simulink model "rtlsdr_datafm_image_audio_Added_Noise"  (R2019a)
settings: Solver=ode45  StartTime=0.0  StopTime=170  RelTol=1e-3  EnableMultiTasking=on
PreLoadFcn:
  | %%%%%%%%%%%%%%%%%%%%%%%%%%%%%%%%%%%%%%%%%%%%%%%%%%%%%%%%%%%%%%%%%%%%%%%%%%%
  | % check to see if Simulink library folder is missing from the MATLAB path %
  | %%%%%%%%%%%%%%%%%%%%%%%%%%%%%%%%%%%%%%%%%%%%%%%%%%%%%%%%%%%%%%%%%%%%%%%%%%%
  | if isempty(strfind(path, 'rtlsdr_book_library'))
  | 
  |     % create error window
  |     fig_error = figure(...
  |         'Name', 'Error: RTL-SDR Book Library',...
  |         'Toolbar','none',...
  |         'MenuBar','none',...
  |         'NumberTitle','off',...
  |         'Resize','off',...
  |         'WindowStyle','modal');
  |     fig_error.Position(3) = 600;
  |     fig_error.Position(4) = 150;
  |     fig_axes = axes(...
  |         'Parent',fig_error,...
  |         'Position',[0,0,1,1],...
  |         'visible','off');
  |     % error message
  |     t_title = text(.05,.8,...
  |         'MISSING DIRECTORIES',...
  |         'FontSize',11.5);
  |     t_body = text(.075,.6,...
  |         [{'Simulink cannot find the  \it{<root>}\rm / \it{rtlsdr\_book\_library}\rm  folder in the \it{MATLAB Path}\rm.'},...
  |         {'Please set the MATLAB path following the instructions given in Exercise 2.4.'}],...
  |         'FontSize',10.5);
  |     % buttons
  |     btn_path = uicontrol(...
  |         'Parent',fig_error,...
  |         'String','Set Path Now',...
  |         'FontSize',10,...
  |         'Callback', 'pathtool; close(fig_error);',...
  |         'Position', [fig_error.Position(3)/2-210, 30, 200, 30]);
  |     btn_abort = uicontrol(...
  |         'Parent',fig_error,...
  |         'String','No thanks',...
  |         'FontSize',10,...
  |         'Callback', 'close(fig_error); abort=1;',...
  |         'Position', [fig_error.Position(3)/2+10, 30, 200, 30]);
  | 
  |     % pause to allow user to interact with error box
  |     uiwait(fig_error);
  | 
  |     % abort simulation
  |     try
  |         if abort==1
  |             set_param(gcs, 'SimulationCommand', 'stop');
  |         end
  |     end
  | 
  |     % if user has set path, allow diagram to be updated
  |     if ~exist('abort','var')
  |         % create error window
  |         fig_update = figure(...
  |             'Name', 'Update Diagram',...
  |             'Toolbar','none',...
  |             'MenuBar','none',...
  |             'NumberTitle','off',...
  |             'Resize','off');
  |         fig_update.Position(3) = 400;
  |         fig_update.Position(4) = 120;
  |         fig_axes = axes(...
  |             'Parent',fig_update,...
  |             'Position',[0,0,1,1],...
  |             'visible','off');
  |         % instruction message
  |         t_body = text(.075,.7,...
  |             'Once you have set the path, update the block diagram',...
  |             'FontSize',10.5);
  |         % button
  |         btn_update = uicontrol(...
  |             'Parent',fig_update,...
  |             'String','Update Block Diagram',...
  |             'FontSize',10,...
  |             'Callback', 'set_param(gcs,''SimulationCommand'',''update''); close(gcf)',...
  |             'Position', [fig_update.Position(3)/2-100, 30, 200, 30]);
  |     end
  | 
  |     % clear error components
  |     clear('fig_error','fig_update','fig_axes','t_title','t_body','btn_path','btn_abort','btn_update','abort');
  | 
  | end
  | %%%%%%%%%%%%%%%%%%%%%%%%%%%%%%%%%%%%%%%%%%%%%%%%%%%%%%%%%%%%%%%%%%%%%%%%%%%
undefined symbols (not defined in the file): dfilt, fdesignblkfcn, frm, gcbh, startfcn_spectrum_analyzer
libraries: dsparch4 x3, simulink x3, dspmlti4 x2, commutil2 x2, simulink_need_slupdate x2, rtlsdr_book_library x2, commrfcorlib x1, commchan3 x1, dspstat3 x1, dspfdesign x1, sdrrlib x1, dspobslib x1
CloseFcn:
  | closefcn_model;
Description:
  | Software, Simulation Examples and Design Exercises Licence Agreement
  | 
  | This license agreement refers to the simulation examples, design exercises and files,
  | and associated software MATLAB and Simulink resources that accompany the book:
  | 
  |      Title: Software Defined Radio using MATLAB & Simulink and the RTL-SDR
  |      Published by Strathclyde Academic Media, 2015
  |      Authored by Robert W. Stewart, Kenneth W. Barlee, Dale S.W. Atkinson,
  |      and Louise H. Crockett
  | 
  | and made available as a download from, www.desktopSDR.com or variously acquired
  | by other means such as via USB storage, cloud storage, disk or any other electronic
  | or optical or magnetic storage mechanism. These files and associated software may
  | be used subject to the terms of agreement of the conditions below:
  | 
  |     Copyright © 2015 Robert W. Stewart, Kenneth W. Barlee, Dale S.W. Atkinson,
  |     and Louise H. Crockett
  |     All rights reserved.
  | 
  | Redistribution and use in source and binary forms, with or without modification, are
  | permitted provided that the following conditions are met:
  | 
  |    1.  Redistributions of source code must retain the above copyright notice, this list of
  |         conditions and the following disclaimer.
  | 
  |    2.  Redistributions in binary form must reproduce the above copyright notice, this
  |         list of conditions and the following disclaimer in the documentation and/or other
  |         materials provided with the distribution.
  | 
  |    3.  Neither the name of the copyright holder nor the names of its contributors may
  |         be used to endorse or promote products derived from this software without
  |         specific prior written permission.
  | 
  |    4.  In all cases, the software is, and all modifications and derivatives of the
  |         software shall be, licensed to you solely for use in conjunction with The
  |         MathWorks, Inc. products and service offerings.
  | 
  | THIS SOFTWARE IS PROVIDED BY THE COPYRIGHT HOLDERS AND CONTRIBUTORS
  | "AS IS" AND ANY EXPRESS OR IMPLIED WARRANTIES, INCLUDING, BUT NOT LIMITED
  | TO, THE IMPLIED WARRANTIES OF MERCHANTABILITY AND FITNESS FOR A
  | PARTICULAR PURPOSE ARE DISCLAIMED. IN NO EVENT SHALL THE COPYRIGHT
  | HOLDER OR CONTRIBUTORS BE LIABLE FOR ANY DIRECT, INDIRECT, INCIDENTAL,
  | SPECIAL, EXEMPLARY, OR CONSEQUENTIAL DAMAGES (INCLUDING, BUT NOT
  | LIMITED TO, PROCUREMENT OF SUBSTITUTE GOODS OR SERVICES; LOSS OF USE,
  | DATA, OR PROFITS; OR BUSINESS INTERRUPTION) HOWEVER CAUSED AND ON ANY
  | THEORY OF LIABILITY, WHETHER IN CONTRACT, STRICT LIABILITY, OR TORT
  | (INCLUDING NEGLIGENCE OR OTHERWISE) ARISING IN ANY WAY OUT OF THE USE
  | OF THIS SOFTWARE, EVEN IF ADVISED OF THE POSSIBILITY OF SUCH DAMAGE.
  | 
  | 
  | Audio Tracks used in Simulations Examples and Design Exercises
  | 
  | The music and vocal files used within the Examples files and software within the book
  | were variously written, arranged, performed, recorded and produced by Garrey Rice,
  | Adam Struth, Jamie Struth, Iain Thistlethwaite and also Marshall Craigmyle who
  | collectively, and individually where appropriate, assert and retain all of their copyright,
  | performance and artistic rights. Permission to use and reproduce this music is
  | granted for all purposes associated with MATLAB and Simulink software and the
  | simulation examples and design exercises files that accompany this book. Requests to
  | use the music for any other purpose should be directed to: info@desktopSDR.com.
  | For information on music track names, full credits, and links to the musicians please
  | refer to www.desktopSDR.com/more/audio.
settings Model: ModifiedByFormat=desktopSDR Team  SimulationMode=accelerator  Creator=desktopSDR Team  LastModifiedBy=desktopSDR Team
settings DataIOCC: SaveFormat=Array  SaveOutput=off  SignalLogging=off  SaveTime=off  ReturnWorkspaceOutputs=off
settings OptimizationCC: LifeSpan=inf
settings DebuggingCC: SolverPrmCheckMsg=warning  AllowSymbolicDim=off  SFUnexpectedBacktrackingDiag=warning  SFNoUnconditionalDefaultTransitionDiag=warning  SFExecutionAtInitializationDiag=none  ArithmeticOperatorsInVariantConditions=warning
settings HardwareCC: ProdBitPerPointer=32  ProdBitPerSizeT=32  ProdBitPerPtrDiffT=32  ProdLargestAtomicFloat=None  ProdIntDivRoundTo=Undefined  ProdEndianess=Unspecified  ProdWordSize=32  ProdHWDeviceType=32-bit Generic
settings ModelReferenceCC: PropagateSignalLabelsOutOfModel=off
settings SFSimCC: SimUseLocalCustomCode=off
settings RTWCC: RTWUseLocalCustomCode=off
settings CodeAppCC: StateflowObjectComments=on
settings GRTTargetCC: TargetLangStandard=C89/C90 (ANSI)  GeneratePreprocessorConditionals=Disable all
settings ConfigComp: CovMetricSettings=dw  CovHtmlReporting=on  CovSaveCumulativeToWorkspaceVar=on  CovSaveSingleToWorkspaceVar=on  CovExternalEMLEnable=off  CovSFcnEnable=off

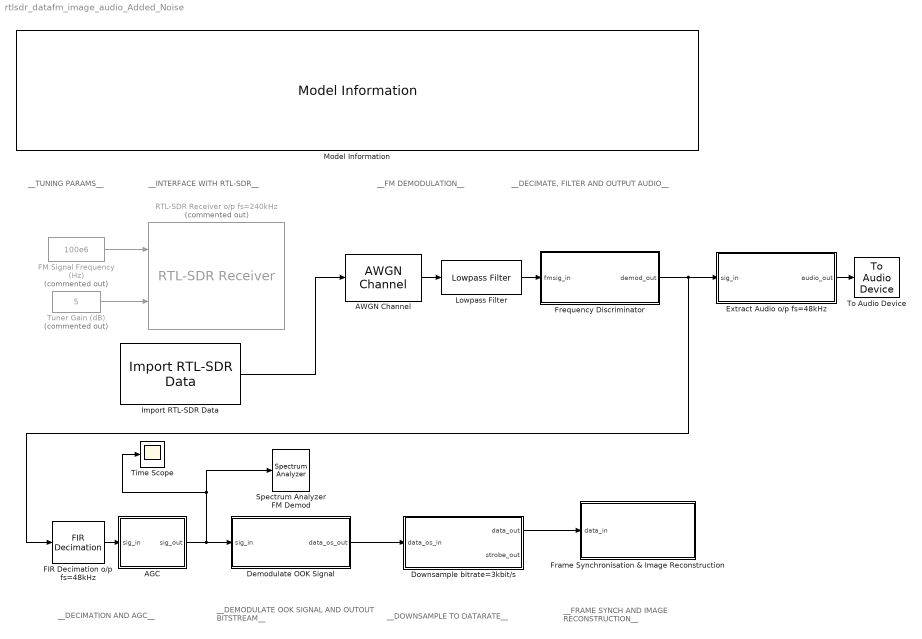
== system rtlsdr_datafm_image_audio_Added_Noise ==
  note: __FRAME SYNCH AND
      | IMAGE RECONSTRUCTION__
  note: __FM DEMODULATION__
  note: __INTERFACE WITH RTL-SDR__
  note: __TUNING PARAMS__
  note: __DECIMATE, FILTER AND OUTPUT AUDIO__
  note: __DECIMATION AND AGC__
  note: __DOWNSAMPLE TO DATARATE__
  note: __DEMODULATE OOK SIGNAL
      | AND OUTOUT BITSTREAM__
  AGC : Subsystem
  AWGN Channel : commchan3/AWGN Channel  InputProcessing=Columns as channels (frame based)  seed=67  noiseMode="Signal to noise ratio  (SNR)"  EbNodB=10  EsNodB=10  SNRdB=10  bitsPerSym=1  Ps=1  Tsym=1  variance=1
      settings: SourceProductName=Communications Toolbox
  Demodulate OOK Signal : Subsystem
  Downsample bitrate=3kbit/s : Subsystem  mask{fs=3e3}
      mask prompts: fs "Data bitrate (bit/s):"
      mask help: This block is used to downsample the received (oversampled) data back to its original bitrate. It comprises of an edge detector and a sampler.
      mask DialogControl DescGroupVar Prompt: Downsampler for Data in FM Signal
  Extract Audio o/p fs=48kHz : Subsystem
  FIR Decimation o/p fs=48kHz : dspmlti4/FIR Decimation  FilterSource=Dialog parameters  h=firpm(150, [0 15e3 20e3 (240e3/2)]/(240e3/2), [1 1 0 0], [1 1],20)  D=5  filtStruct=Direct form  FilterObject=Hm_firdecim  InputProcessing=Columns as channels (frame based)  framing=Allow multirate processing  inputOffset=0  outputBufInitCond=0  roundingMode=Floor  overflowMode=off  firstCoeffDataTypeStr=Inherit: Same word length as input  firstCoeffMin=[]  firstCoeffMax=[]  firstCoeffLastDataTypeStr=Inherit: Same word length as input  outputDataTypeStr=Inherit: Same as accumulator  outputMin=[]  outputMax=[]  outputLastDataTypeStr=Inherit: Same as accumulator
  "FM Signal Frequency (Hz) " : Constant  Commented=on  Value=100e6
  Frame Synchronisation & Image Reconstruction : Subsystem  mask(Receiver Parameter Settings){binary_len=8}
      mask prompts: binary_len "Image Pixel Bit Depth"
      mask help: The subsystem implements frame synchronisation to re-frame the received data back to its original frame structure. The preamble is then removed before the remaining header and payload data are used to recover and reconstruct the transmitted image.
      mask init:
      | try 
      |     image_receive;
      | catch ME
      |     if(strcmp(ME.identifier,'MATLAB.UndefinedFunction'))
      |         error('Unable to find "image_receive.m".');
      |     end
      |     rethrow(ME);
      | end
      mask Callback binary_len:
      | try
      |     image_receive;
      | end
  Frequency Discriminator : Subsystem
  Import RTL-SDR Data : rtlsdr_book_library/Additional Tools/Import RTL-SDR Data  filename=datafm_image_audio.mat  frm_size=4096  data_type=single
      settings: SourceProductName=RTL-SDR Book Library
  Lowpass Filter : dspfdesign/Lowpass Filter  FilterType=FIR  DesignForMinimumOrder=on  FilterOrder=50  PassbandFrequency=5e3  StopbandFrequency=80e3  PassbandRipple=0.1  StopbandAttenuation=80  InheritSampleRate=off  SampleRate=240e3  SimulateUsing=Interpreted execution  roundingMode=Floor  coeffsDataTypeStr=fixdt(1,16)
  Model Information : rtlsdr_book_library/Additional Tools/Model Information/Model Information
      settings: SourceProductName=RTL-SDR Book Library
  RTL-SDR Receiver o/p fs=240kHz : sdrrlib/RTL-SDR Receiver  Commented=on  IPAddress=0  CenterFrequencySource=Input port  CenterFrequency=433.9e6  GainSource=Input port  Gain=15  ADCRate=240e3  FrequencyCorrection=0  LostSamplesOutputPort=off  LatencyOutputPort=off  OutputDataType=single  FrameLength=4096  EnableBurstMode=off  NumFramesInBurst=20  sobjType=sdrr.internal.SDRRTLReceiverSL  dataUDPPort=-1  ctrlUDPPort=-1  subDeviceList=nosubdev  sdrBlockType=SDRBlockTypeSLT.SDRRxBlock  requester=UNUSED_BY_SFCN  sdrExecutionMode=SDRExecutionModeSLT.ExecModeHW  BypassUserLogic=off  DecimatorSelect=DDC decimator  SourceSelect=RF data  SineAmplitude=16000  EnableInternalClock=off  BypassIQBalance=off  IFBandwidth=40e6  ADCRateSource=Dialog  IntermediateFrequency=0  DecimationFactorSource=Dialog  DecimationFactor=512  RFFrequencyIsTunable=logical(1)  SampleTime=(4096)/(240e3)  IFBandwidthSource=Dialog  SineFrequency=30000  BypassDCBlockingFilter=off  IntermediateFrequencySource=Dialog  IQBalanceCoefficients=64  SkipAllHardwareResetAndInitialization=off  EnableIQCalibrationTable=on  CacheIQCalibrationTable=off  EnableOffsetTuning=off  EnableRTLAGC=off  EnableTestMode=off  EnableTunerAGC=off  FrequencyCorrectionSource=Dialog  NumMLBuffers=128  NumUSBBuffers=16  RTLCrystalFrequency=28800000  TunerCrystalFrequency=28800000
      settings: SourceProductName=Communications Toolbox Support Package for RTL-SDR Radio  SourceProductBaseCode=RTLSDR
  Spectrum Analyzer FM Demod : SpectrumAnalyzer  StartFcn=startfcn_spectrum_analyzer;
  Time Scope : Scope
      settings: StartFcn=startfcn_time_scope
  To Audio Device : dspobslib/To Audio Device  deviceName=Default  inheritSampleRate=on  sampleRate=44100  deviceDatatype=Determine from input data type  autoBufferSize=on  bufferSize=4096  queueDuration=1.0  defaultOutputChannelMapping=on  outputChannelMapping=1:2  outputNumUnderrunSamples=off
      settings: SourceProductName=DSP System Toolbox  SourceProductBaseCode=DS
  Tuner Gain (dB) : Constant  Commented=on  Value=5
  wires:
  Tuner Gain (dB)/1 -> RTL-SDR Receiver o/p fs=240kHz/2
  "FM Signal Frequency (Hz) "/1 -> RTL-SDR Receiver o/p fs=240kHz/1
  Extract Audio o/p fs=48kHz/1(audio_out) -> To Audio Device/1
  Downsample bitrate=3kbit/s/1(data_out) -> Frame Synchronisation & Image Reconstruction/1(data_in)
  FIR Decimation o/p fs=48kHz/1 -> AGC/1(sig_in)
  Frequency Discriminator/1(demod_out) -> Extract Audio o/p fs=48kHz/1(sig_in), FIR Decimation o/p fs=48kHz/1
  Demodulate OOK Signal/1(data_os_out) -> Downsample bitrate=3kbit/s/1(data_os_in)
  AGC/1(sig_out) -> Demodulate OOK Signal/1(sig_in), Time Scope/1, Spectrum Analyzer FM Demod/1
  AWGN Channel/1 -> Lowpass Filter/1
  Import RTL-SDR Data/1 -> AWGN Channel/1
  Lowpass Filter/1 -> Frequency Discriminator/1(fmsig_in)

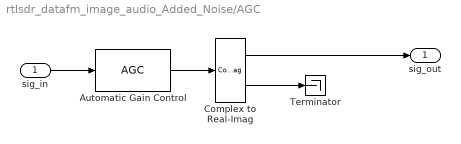
== system rtlsdr_datafm_image_audio_Added_Noise/AGC ==
  sig_in : Inport
  Automatic Gain Control : commrfcorlib/AGC  LegacyMode=off  DetectorMethod=Rectifier  LoopMethod=Linear  UpdatePeriod=128  StepSize=0.03  AdaptationStepSize=(0.03)/(128)  DesiredOutputPower=1  AveragingLength=128  MaximumGain=20  MaxPowerGain=20  GainOutputPort=off  InputPowerOutputPort=off  SimulateUsing=Code generation
      settings: SourceProductName=Communications Toolbox
  Complex to Real-Imag : ComplexToRealImag
  Terminator : Terminator
  sig_out : Outport
  wires:
  Complex to Real-Imag/1 -> sig_out/1
  Automatic Gain Control/1 -> Complex to Real-Imag/1
  sig_in/1 -> Automatic Gain Control/1
  Complex to Real-Imag/2 -> Terminator/1

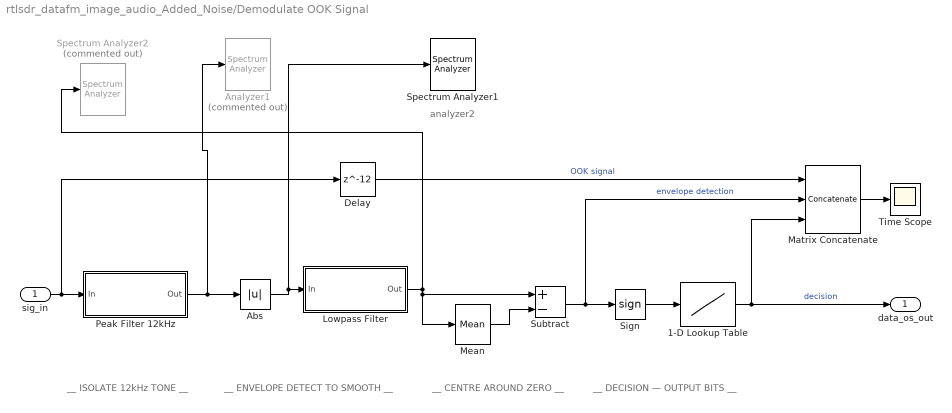
== system rtlsdr_datafm_image_audio_Added_Noise/Demodulate OOK Signal ==
  note: analyzer2
  note: __ ISOLATE 12kHz TONE __
  note: __ ENVELOPE DETECT TO SMOOTH __
  note: __ CENTRE AROUND ZERO __
  note: __ DECISION — OUTPUT BITS __
  sig_in : Inport
  " Analyzer1" : SpectrumAnalyzer  Commented=on
  1-D Lookup Table : Lookup_n-D  NumberOfTableDimensions=1  BreakpointsForDimension1=[-1,0,1]  Table=[0,0,1]  InternalRulePriority=Speed  RndMeth=Simplest  InputSameDT=on
  Abs : Abs
  Delay : Delay  DelayLength=12  InputProcessing=Columns as channels (frame based)
  Lowpass Filter : Subsystem  DialogController=fdesignblkfcn  InitFcn=fdesignblkfcn(gcbh, {'InitFcn'});  mask(Lowpass Filter){}
      mask help: Design a lowpass filter
      settings: CopyFcn=fdesignblkfcn(gcbh, {'CopyFcn'});
      mask Help: helpview(mapfilelocation('dsp'), 'dsplowpassfilter');
      mask Display: disp('Lowpass')
  Matrix Concatenate : Concatenate  NumInputs=3  Mode=Multidimensional array  ConcatenateDimension=2
  Mean : dspstat3/Mean  run=off  InputProcessing=Columns as channels (frame based)  reset_popup=None  directionMode=Each column  dimension=1  roiEnable=off  roiType=Rectangles  roiPortion=Entire ROI  roiOutput=Individual statistics for each ROI  roiFlag=off  roundingMode=Floor  overflowMode=off  outputDataTypeStr=Inherit: Same as accumulator  outputMin=[]  outputMax=[]  outputLastDataTypeStr=Inherit: Same as accumulator
  Peak Filter 12kHz : Subsystem  DialogController=fdesignblkfcn  InitFcn=fdesignblkfcn(gcbh, {'InitFcn'});  mask(Peak/Notch Filter){}
      mask help: Design a peak/notch filter
      settings: CopyFcn=fdesignblkfcn(gcbh, {'CopyFcn'});
      mask Help: helpview(mapfilelocation('dsp'), 'dsppeaknotchfilter');
      mask Display: disp('Peak-Notch');
  Sign : Signum
  Spectrum Analyzer1 : SpectrumAnalyzer
  Spectrum Analyzer2 : SpectrumAnalyzer  Commented=on
  Subtract : Sum  Inputs=+-
  Time Scope : Scope
      settings: StartFcn=startfcn_time_scope
  data_os_out : Outport
  wires:
  Abs/1 -> Spectrum Analyzer1/1, Lowpass Filter/1(In)
  Lowpass Filter/1(Out) -> Spectrum Analyzer2/1, Subtract/1, Mean/1
  Peak Filter 12kHz/1(Out) -> " Analyzer1"/1, Abs/1
  Sign/1 -> 1-D Lookup Table/1
  1-D Lookup Table/1 -> Matrix Concatenate/3, data_os_out/1  "decision"
  Subtract/1 -> Matrix Concatenate/2, Sign/1  "envelope detection"
  Mean/1 -> Subtract/2
  sig_in/1 -> Peak Filter 12kHz/1(In), Delay/1
  Matrix Concatenate/1 -> Time Scope/1
  Delay/1 -> Matrix Concatenate/1  "OOK signal"

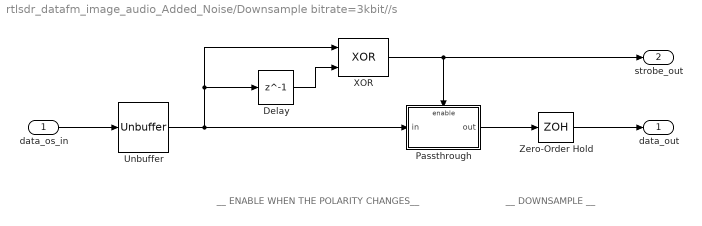
== system rtlsdr_datafm_image_audio_Added_Noise/Downsample bitrate=3kbit//s ==
  note: __ DOWNSAMPLE __
  note: __ ENABLE WHEN THE POLARITY CHANGES__
  data_os_in : Inport
  Delay : Delay  DelayLength=1  InitialCondition=0
  Passthrough : Subsystem
  Unbuffer : Unbuffer
  XOR : Logic  Operator=XOR  IconShape=distinctive  AllPortsSameDT=off  OutDataTypeStr=boolean
  Zero-Order Hold : ZeroOrderHold  SampleTime=1/fs
  data_out : Outport
  strobe_out : Outport  Port=2
  wires:
  Zero-Order Hold/1 -> data_out/1
  Unbuffer/1 -> Delay/1, XOR/1, Passthrough/1(in)
  Delay/1 -> XOR/2
  XOR/1 -> strobe_out/1, Passthrough/Enable
  Passthrough/1(out) -> Zero-Order Hold/1
  data_os_in/1 -> Unbuffer/1

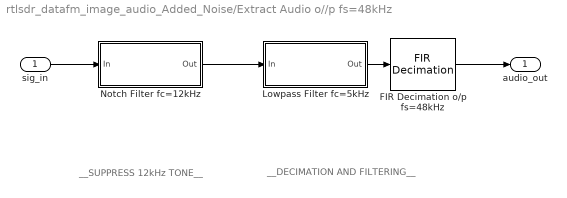
== system rtlsdr_datafm_image_audio_Added_Noise/Extract Audio o//p fs=48kHz ==
  note: __SUPPRESS 12kHz TONE__
  note: __DECIMATION AND FILTERING__
  sig_in : Inport
  FIR Decimation o/p fs=48kHz : dspmlti4/FIR Decimation  FilterSource=Dialog parameters  h=firpm(150, [0 15e3 20e3 (240e3/2)]/(240e3/2), [1 1 0 0], [1 1],20)  D=5  filtStruct=Direct form  FilterObject=Hm_firdecim  InputProcessing=Columns as channels (frame based)  framing=Allow multirate processing  inputOffset=0  outputBufInitCond=0  roundingMode=Floor  overflowMode=off  firstCoeffDataTypeStr=Inherit: Same word length as input  firstCoeffMin=[]  firstCoeffMax=[]  firstCoeffLastDataTypeStr=Inherit: Same word length as input  outputDataTypeStr=Inherit: Same as accumulator  outputMin=[]  outputMax=[]  outputLastDataTypeStr=Inherit: Same as accumulator
  Lowpass Filter fc=5kHz : Subsystem  DialogController=fdesignblkfcn  InitFcn=fdesignblkfcn(gcbh, {'InitFcn'});  mask(Lowpass Filter){}
      mask help: Design a lowpass filter
      settings: CopyFcn=fdesignblkfcn(gcbh, {'CopyFcn'});
      mask Help: helpview(mapfilelocation('dsp'), 'dsplowpassfilter');
      mask Display: disp('Lowpass')
  Notch Filter fc=12kHz : Subsystem  DialogController=fdesignblkfcn  InitFcn=fdesignblkfcn(gcbh, {'InitFcn'});  mask(Peak/Notch Filter){}
      mask help: Design a peak/notch filter
      settings: CopyFcn=fdesignblkfcn(gcbh, {'CopyFcn'});
      mask Help: helpview(mapfilelocation('dsp'), 'dsppeaknotchfilter');
      mask Display: disp('Peak-Notch');
  audio_out : Outport
  wires:
  sig_in/1 -> Notch Filter fc=12kHz/1(In)
  FIR Decimation o/p fs=48kHz/1 -> audio_out/1
  Lowpass Filter fc=5kHz/1(Out) -> FIR Decimation o/p fs=48kHz/1
  Notch Filter fc=12kHz/1(Out) -> Lowpass Filter fc=5kHz/1(In)

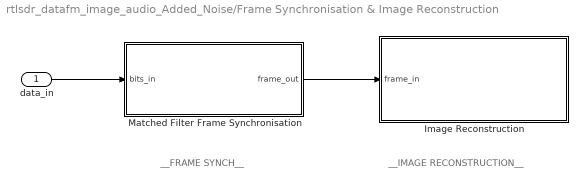
== system rtlsdr_datafm_image_audio_Added_Noise/Frame Synchronisation & Image Reconstruction ==
  note: __FRAME SYNCH__
  note: __IMAGE RECONSTRUCTION__
  data_in : Inport
  Image Reconstruction : Subsystem  AncestorBlock=rtlsdr_book_library/Data Comms Sources and Sinks/Image Reconstruction  InitFcn=|  mask(Image Reconstruction){}
      | % create figure window, plot empty image then hide
      | hfig = figure;
      | imshow(uint8(zeros(100,100)),'InitialMagnification',250);
      | hfig.Visible = 'off';
      mask help: This block will receive and process frames of image data. When the full image has been receieved, the simulation will pause, and the image will be displayed.
      settings: CloseFcn=clear('hfig','hax');
      settings: PauseFcn=|
      | % set current figure to handle
      | set(0,'CurrentFigure',hfig);
      | 
      | % make plot visible if not already
      | hfig.Visible = 'on'
      | 
      | % plot image
      | imshow(uint8(image),'InitialMagnification',250);
      | 
      | % configure image figure window
      | hfig.MenuBar = 'none';
      | hfig.ToolBar = 'none';
      | hfig.Resize = 'off';
      | hfig.Name = 'Received Image';
      | hfig.NumberTitle = 'off';
      | hfig.Position = [hfig.Position(1)+45,hfig.Position(2)+3,330,335];
      | hax = gca;
      | hax.Units = 'pixels';
      | hax.Position = [40,45,250,250];
      | 
      | % resume simulation
      | set_param(bdroot, 'SimulationCommand', 'continue')
  Matched Filter Frame Synchronisation : Subsystem
  wires:
  data_in/1 -> Matched Filter Frame Synchronisation/1(bits_in)
  Matched Filter Frame Synchronisation/1(frame_out) -> Image Reconstruction/1(frame_in)

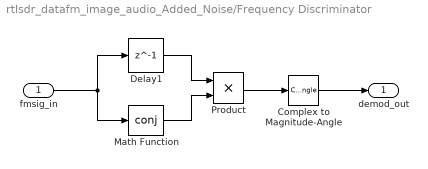
== system rtlsdr_datafm_image_audio_Added_Noise/Frequency Discriminator ==
  fmsig_in : Inport
  Complex to Magnitude-Angle : ComplexToMagnitudeAngle  Output=Angle
  Delay1 : Delay  DelayLength=1  InitialCondition=0  InputProcessing=Columns as channels (frame based)
  Math Function : Math  Operator=conj  SaturateOnIntegerOverflow=on
  Product : Product
  demod_out : Outport
  wires:
  fmsig_in/1 -> Delay1/1, Math Function/1
  Delay1/1 -> Product/1
  Product/1 -> Complex to Magnitude-Angle/1
  Math Function/1 -> Product/2
  Complex to Magnitude-Angle/1 -> demod_out/1

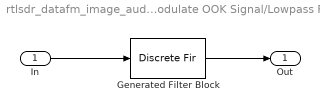
== system rtlsdr_datafm_image_audio_Added_Noise/Demodulate OOK Signal/Lowpass Filter ==
  In : Inport
  Generated Filter Block : DiscreteFir  Tag=BlockMethodSubSystem  Coefficients=[-0.0011039148487577415 -0.00421743301345689232 -0.00335085420937103343 -0.00293490474113965215 0.000149394565669530707 0.00462387135842150937 0.00932167040158395251 0.0119561970091274748 0.0103483768398457583 0.00331727080415413975 -0.00834682879990942053 -0.0214777410399142228 -0.0309894580889876689 -0.0311578834932403487 -0.0174838287634073164 0.011487187147605004 0.0530812806303288462 0.100597979734233872 0.144734798152597016 0.175988173448287738 0.187278728240815456 0.175988173448287738 0.144734798152597016 0.100597979734233872 0.0530812806303288462 0.011487187147605004 -0.0174838287634073164 -0.0311578834932403487 -0.0309894580889876689 -0.0214777410399142228 -0.00834682879990942053 0.00331727080415413975 0.0103483768398457583 0.0119561970091274748 0.00932167040158395251 0.00462387135842150937 0.000149394565669530707 -0.00293490474113965215 -0.00335085420937103343 -0.00421743301345689232 -0.0011039148487577415]  InputProcessing=Columns as channels (frame based)
  Out : Outport
  wires:
  Generated Filter Block/1 -> Out/1
  In/1 -> Generated Filter Block/1

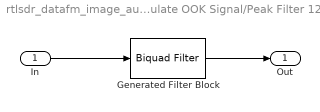
== system rtlsdr_datafm_image_audio_Added_Noise/Demodulate OOK Signal/Peak Filter 12kHz ==
  In : Inport
  Generated Filter Block : dsparch4/Biquad Filter  Tag=BlockMethodSubSystem  FilterSource=Dialog parameters  CoeffSource=Specify via dialog  FilterObject=BQF  IIRFiltStruct=Direct form II  BiQuadCoeffs=[0.500000000000000222 0 -0.500000000000000222 1 0 0.546041311705949939]  ScaleValues=[0.453958688294050006;1]  IC=0  ICnum=0  ICden=0  a0Flag=Warning  optimizeScaleValues=off  ScaleValueMode=Specify via input port (g)  InputProcessing=Columns as channels (frame based)  roundingMode=Floor  overflowMode=off  scaleValueFracLength=14  denProdOutputFracLength=30  denAccumFracLength=30  secondMemoryFracLength=15
      settings: SourceProductName=DSP System Toolbox
  Out : Outport
  wires:
  In/1 -> Generated Filter Block/1
  Generated Filter Block/1 -> Out/1

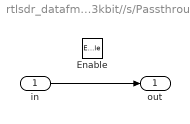
== system rtlsdr_datafm_image_audio_Added_Noise/Downsample bitrate=3kbit//s/Passthrough ==
  in : Inport
  Enable : EnablePort
  out : Outport
  wires:
  in/1 -> out/1

== system rtlsdr_datafm_image_audio_Added_Noise/Extract Audio o//p fs=48kHz/Lowpass Filter fc=5kHz ==
  In : Inport
  Generated Filter Block : dsparch4/Biquad Filter  Tag=BlockMethodSubSystem  FilterSource=Dialog parameters  CoeffSource=Specify via dialog  FilterObject=dfilt.df2tsos([1 0.3 0.4],[1 0.1 0.2])  IIRFiltStruct=Direct form II  BiQuadCoeffs=[0.0014662393146652132 0.0029324786293304264 0.0014662393146652132 1 -1.966487213158906 0.98042551630274088;0.0022920241445179498 0.0045840482890358997 0.0022920241445179498 1 -1.9364922852784932 0.9502179867868954;0.0030462749460832615 0.006092549892166523 0.0030462749460832615 1 -1.9082335044404777 0.92175890998399401;0.0037193449217970583 0.0074386898435941165 0.0037193449217970583 1 -1.882082606511571 0.89542265659466191;0.0043036790546654565 0.0086073581093309131 0.0043036790546654565 1 -1.8583493452763198 0.87152117591334699;0.0047934341700202826 0.0095868683400405653 0.0047934341700202826 1 -1.8372871407642493 0.85030968419035424;0.0051785274900342463 0.010357054980068493 0.0051785274900342463 1 -1.819099402132154 0.83199303233021527;0.0054523704074212146 0.010904740814842429 0.0054523704074212146 1 -1.8039459107783395 0.81673213424893054;0.005590224938626656 0.011180449877253312 0.005590224938626656 1 -1.7919488018634986 0.80464999079138577;0.0054805240423490848 0.01096104808469817 0.0054805240423490848 1 -1.783197814344097 0.79583697697654865;0.0037737208845104188 0.0075474417690208377 0.0037737208845104188 1 -1.7777545856157935 0.79035516708097953;0.0031475426526353378 0.0062950853052706757 0.0031475426526353378 1 -1.7756558469630193 0.78824155273749852;0.0031542303018931022 0.0063084606037862043 0.0031542303018931022 1 -1.7762857689079308 0.78887593951847212;0.0031668170202996393 0.0063336340405992786 0.0031668170202996393 1 -1.7800598801798011 0.7926768013873734;0.0031852162333163569 0.0063704324666327139 0.0031852162333163569 1 -1.7871630750369847 0.79983034311818335;0.0032092946571374292 0.0064185893142748585 0.0032092946571374292 1 -1.7975464959615994 0.81028736089486497;0.0032388656379085386 0.0064777312758170771 0.0032388656379085386 1 -1.8111349255052718 0.82397210413382149;0.0032736806555420657 0.0065473613110841314 0.0032736806555420657 1 -1.8278230273400591 0.84077848989169335;0.0033134193124529925 0.0066268386249059849 0.0033134193124529925 1 -1.8474705515172725 0.86056527413944062;0.0033576782919589876 0.0067153565839179752 0.0033576782919589876 1 -1.8698966847064717 0.88315036195628382;0.0034059599823703102 0.0068119199647406203 0.0034059599823703102 1 -1.8948738189724748 0.90830453214031059;0.0034576617167602634 0.0069153234335205269 0.0034576617167602634 1 -1.9221211318896212 0.93574497181910243;0.0016067126669943627 0.0032134253339887254 0.0016067126669943627 1 -1.9512985141080388 0.96512916097507984;0.00080552544491969372 0.0016110508898393874 0.00080552544491969372 1 -1.9820015389165753 0.99604980635310192;0.0016828305703076845 0.003365661140615369 0.0016828305703076845 1 -1.9588485075461843 0.97273266815924442;0.0025064364169543859 0.0050128728339087717 0.0025064364169543859 1 -1.9292491998705552 0.94292356297236302;0.0032651962074720033 0.0065303924149440066 0.0032651962074720033 1 -1.9014850466339253 0.91496261965148828;0.0039502465940013855 0.0079004931880027711 0.0039502465940013855 1 -1.87591182318419 0.88920813525155573;0.0045523843762476958 0.0091047687524953916 0.0045523843762476958 1 -1.8528246319757433 0.8659573038894125;0.005055714640913209 0.010111429281826418 0.005055714640913209 1 -1.8324637859255974 0.84545214180069195;0.0054808525254435277 0.010961705050887055 0.0054808525254435277 1 -1.8150211977296618 0.82788592194304933;0.0058118949086395115 0.011623789817279023 0.0058118949086395115 1 -1.800646700304964 0.81340953923717341;0.0060459949514982715 0.012091989902996543 0.0060459949514982715 1 -1.789453871767567 0.80213737683167541;0.0051564308167370808 0.010312861633474162 0.0051564308167370808 1 -1.781525064055334 0.79415237036832775;0.0031468761340607944 0.0062937522681215888 0.0031468761340607944 1 -1.7769154336553292 0.78951006727893736;0.0031520029214611171 0.0063040058429222343 0.0031520029214611171 1 -1.7758658494881789 0.78845304374365988;0.0031631212822456067 0.0063262425644912135 0.0031631212822456067 1 -1.7788028792111099 0.79141089089695449;0.0031800779436629845 ...(+1046 chars)]  ScaleValues=[0.0023105936150123589;1;1;1;1;1;1;1;1;1;1;1;1;1;1;1;1;1;1;1;1;1;1;1;1;1;1;1;1;1;1;1;1;1;1;1;1;1;1;1;1;1;1;1;1;1;1;1]  IC=0  ICnum=0  ICden=0  a0Flag=Warning  optimizeScaleValues=off  ScaleValueMode=Specify via input port (g)  InputProcessing=Columns as channels (frame based)  roundingMode=Floor  overflowMode=off  scaleValueFracLength=14  denProdOutputFracLength=30  denAccumFracLength=30  secondMemoryFracLength=15
      settings: SourceProductName=DSP System Toolbox
  Out : Outport
  wires:
  Generated Filter Block/1 -> Out/1
  In/1 -> Generated Filter Block/1

== system rtlsdr_datafm_image_audio_Added_Noise/Extract Audio o//p fs=48kHz/Notch Filter fc=12kHz ==
  In : Inport
  Generated Filter Block : dsparch4/Biquad Filter  Tag=BlockMethodSubSystem  FilterSource=Dialog parameters  CoeffSource=Specify via dialog  FilterObject=BQF  IIRFiltStruct=Direct form II  BiQuadCoeffs=[1.05146229050548512 -2 1.05146209890108522 1 -1.8906743662652028 0.982176158478403227;1.05146235262899834 -2 1.0514621549175398 1 -1.87834367169647365 0.981140680218305361]  ScaleValues=[0.00535108106216475744;1;165.93249752525395]  IC=0  ICnum=0  ICden=0  a0Flag=Warning  optimizeScaleValues=off  ScaleValueMode=Specify via input port (g)  InputProcessing=Columns as channels (frame based)  roundingMode=Floor  overflowMode=off  scaleValueFracLength=14  denProdOutputFracLength=30  denAccumFracLength=30  secondMemoryFracLength=15
      settings: SourceProductName=DSP System Toolbox
  Out : Outport
  wires:
  Generated Filter Block/1 -> Out/1
  In/1 -> Generated Filter Block/1

== system rtlsdr_datafm_image_audio_Added_Noise/Frame Synchronisation & Image Reconstruction/Image Reconstruction ==
  frame_in : Inport
  Binary Length of Pixel : Constant  Value=frm.binary_len  VectorParams1D=off  OutDataTypeStr=single  FramePeriod=-1
  Image Reconstruction : MATLAB Function  TreatAsAtomicUnit=on
  wires:
  Binary Length of Pixel/1 -> Image Reconstruction/2(binary_len)
  frame_in/1 -> Image Reconstruction/1(frame_in)

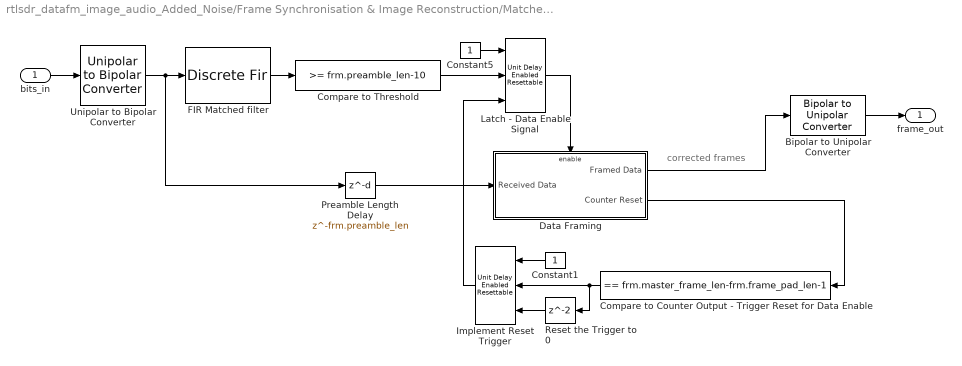
== system rtlsdr_datafm_image_audio_Added_Noise/Frame Synchronisation & Image Reconstruction/Matched Filter Frame Synchronisation ==
  note: corrected frames
  bits_in : Inport
  Bipolar to Unipolar Converter : commutil2/Bipolar to Unipolar Converter  M=2  polarity=Positive  dataType=Inherit via internal rule
      settings: SourceProductName=Communications Toolbox  SourceProductBaseCode=CM
  Compare to Counter Output - Trigger Reset for Data Enable : simulink/Logic and Bit Operations/Compare To Constant  relop===  const=frm.master_frame_len-frm.frame_pad_len-1  OutDataTypeStr=boolean
  Compare to Threshold : simulink/Logic and Bit Operations/Compare To Constant  relop=>=  const=frm.preamble_len-10  OutDataTypeStr=boolean
  Constant1 : Constant
  Constant5 : Constant
  Data Framing : Subsystem
  FIR Matched filter : DiscreteFir  Coefficients=frm.filter_coeff  InputProcessing=Columns as channels (frame based)
  Implement Reset Trigger : simulink_need_slupdate/Unit Delay Enabled Resettable  vinit=0  tsamp=-1
      settings: SourceProductName=Simulink  SourceProductBaseCode=SL
  Latch - Data Enable Signal : simulink_need_slupdate/Unit Delay Enabled Resettable  vinit=0  tsamp=-1
      settings: SourceProductName=Simulink  SourceProductBaseCode=SL
  Preamble Length Delay : Delay  DelayLength=frm.preamble_len  DelayLengthUpperLimit=10000  InitialCondition=1
  Reset the Trigger to 0 : Delay  DelayLengthUpperLimit=10000  InitialCondition=0
  Unipolar to Bipolar Converter : commutil2/Unipolar to Bipolar Converter  M=2  polarity=Positive  dataType=Inherit via internal rule
      settings: SourceProductName=Communications Toolbox
  frame_out : Outport
  wires:
  Unipolar to Bipolar Converter/1 -> FIR Matched filter/1, Preamble Length Delay/1
  Bipolar to Unipolar Converter/1 -> frame_out/1
  Data Framing/2(Counter Reset) -> Compare to Counter Output - Trigger Reset for Data Enable/1
  Reset the Trigger to 0/1 -> Implement Reset Trigger/3
  FIR Matched filter/1 -> Compare to Threshold/1
  Preamble Length Delay/1 -> Data Framing/1(Received Data)
  Data Framing/1(Framed Data) -> Bipolar to Unipolar Converter/1
  Compare to Counter Output - Trigger Reset for Data Enable/1 -> Implement Reset Trigger/2, Reset the Trigger to 0/1
  Compare to Threshold/1 -> Latch - Data Enable Signal/2
  Constant1/1 -> Implement Reset Trigger/1
  bits_in/1 -> Unipolar to Bipolar Converter/1
  Constant5/1 -> Latch - Data Enable Signal/1
  Latch - Data Enable Signal/1 -> Data Framing/Enable
  Implement Reset Trigger/1 -> Latch - Data Enable Signal/3

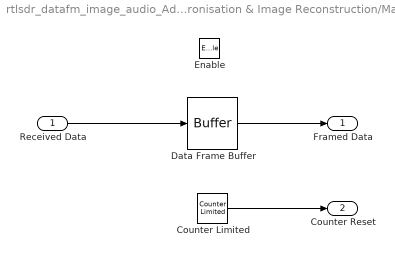
== system rtlsdr_datafm_image_audio_Added_Noise/Frame Synchronisation & Image Reconstruction/Matched Filter Frame Synchronisation/Data Framing ==
  Received Data : Inport
  Enable : EnablePort
  Counter Limited : simulink/Sources/Counter Limited  uplimit=frm.master_frame_len-frm.frame_pad_len-1  tsamp=-1
  Data Frame Buffer : Buffer  N=frm.master_frame_len-frm.frame_pad_len
  Framed Data : Outport
  Counter Reset : Outport  Port=2
  wires:
  Received Data/1 -> Data Frame Buffer/1
  Data Frame Buffer/1 -> Framed Data/1
  Counter Limited/1 -> Counter Reset/1

== matlab function rtlsdr_datafm_image_audio_Added_Noise/Frame Synchronisation & Image Reconstruction/Image Reconstruction/Image Reconstruction ==
  data: frame_in input; binary_len input
%% Image Transfer: Image Reconstruction
% This function is used to process received frames of data and rebuild the
% image that has been transferred. Once the appropriate number of frames
% has been retrieved, the image is then plotted in a figure for the user to
% observe.

function message_decoder_img_transfer(frame_in, binary_len)

%% FUNCTION SETUP
% functions that cannot be compiled
coder.extrinsic('assignin')
coder.extrinsic('get_param')
coder.extrinsic('set_param')
coder.extrinsic('num2str')
coder.extrinsic('bdroot')
coder.extrinsic('gcs')
coder.extrinsic('disp')

%% PROTOCOL PARAMETERS
% make frame length persistent across function calls
persistent frame_len;
% initialise variable on first call to function
if isempty(frame_len)
    frame_len = 1000;                                                      % total length of a frame
end

%% IMAGE RECONSTRUCTION PARAMETERS
% make variables persistent across function calls
persistent image seq_num_storage valid_seq_num prev_seqnum sequence_num...
    initial_op_flag seqnum_lock seqnum_countenable;

% initialise variables
img_rx = 0;                                                                % variable that will hold each input frame
data_len = 0;                                                              % variable to store data length of each frame
header_len = 0;                                                            % variable to store header length of each frame
img_pixels_x = 100;                                                        % default value for image width
img_pixels_y = 100;                                                        % default value for image height

% initialise persistent variables on first call to function
if isempty(initial_op_flag)
    initial_op_flag = 0;                                                   % initialise output flag for information message to print
end
if isempty(image)
    image = zeros(img_pixels_x,img_pixels_y);                              % initialise image storage variable
    image(1:img_pixels_x,1:img_pixels_y) = uint8(255);                     % set matrix values to 255 - making default matrix a white background
end
if isempty(seq_num_storage)
    seq_num_storage = zeros(1,img_pixels_x);                               % initialise sequence number storage
end
if isempty(valid_seq_num)
    valid_seq_num = 1;                                                     % set valid sequence number flag high
end
if isempty(prev_seqnum)
    prev_seqnum = zeros(1,4);                                              % initialise previous sequence number vector for storage of past values
end
if isempty(sequence_num)
    sequence_num = 1;                                                      % initialise sequence number to store individual frame's sequence number
end
if isempty(seqnum_lock)
    seqnum_lock = 0;                                                       % set sequence number lock low
end
if isempty(seqnum_countenable)
    seqnum_countenable = 0;                                                % set sequence number count enable low
end

% assert specific variables for code generation
assert (data_len <= frame_len);
assert (header_len <= frame_len);
assert (img_rx <= frame_len);

% provide bounds for size of variables 'payload' and 'pixel_column'
coder.varsize ('payload', 1000);
coder.varsize ('pixel_column', [1 100]);

%% HEADER PARAMETERS
persistent seq_num_bit_len end_flag_bit_len header_bit_len payload_bit_len pad_bit_len;
if isempty(seq_num_bit_len)
    seq_num_bit_len = 8;                                                   % # of bits in header - frame sequence number length
end
if isempty(end_flag_bit_len)
    end_flag_bit_len = 1;                                                  % # of bits in header - end packet flag length
end
if isempty(header_bit_len)
    header_bit_len = 8;                                                    % # of bits in header - header length
end
if isempty(payload_bit_len)
    payload_bit_len = 10;                                                  % # of bits in header - payload length
end
if isempty(pad_bit_len)
    pad_bit_len = 9;                                                       % # of bits in header - padding length
end

%% Frame Header Structure
%-------------------------------------------------------------------------%
% Frame Header- [Preamble, sequence number, end flag, header length,
%                payload length, padding length]
%-------------------------------------------------------------------------%

% set the preamble in unipolar form - used at the beginning of each frame
preamble = [1,1,1,1,1,1,1,1,1,1,1,1,1,1,1,0,0,0,0,0,0,1,1,1,1,1,1,0,0,0,1,1,1,0,0,0,1,1,1];
preamble_len = length(preamble);                                           % calculate decimal length of the preamble sequence
preamble_pad_len = rem(preamble_len,2);                                    % determine length of preamble padding

% determine the starting index positions for the fields of the header
seq_num_pos = preamble_len + preamble_pad_len+1;                           % sequence number starts after the preamble
end_flag_pos = seq_num_pos + seq_num_bit_len;                              % end flag (indicating last frame) starts after the sequence number
header_len_pos = end_flag_pos + end_flag_bit_len;                          % header length starts after the end flag
payload_len_pos = header_len_pos + header_bit_len;                         % payload length starts after the header length
pad_len_pos = payload_len_pos + payload_bit_len;                           % padding length starts after the payload length

% typecast the input frame to uint8 and store in 'img_rx'
img_rx = uint8(frame_in);

%-------------------------------------------------------------------------%
% Store and use previous sequence numbers to obtain a sequence lock signal

% prev_seqnum stores the current and last three sequence numbers
for i = 4:-1:2
    prev_seqnum(i) = prev_seqnum(i-1);                                     % shift previous sequence numbers in register - oldest shifted out
end
prev_seqnum(1) = sequence_num;                                             % store current sequence number before next current value is obtained

if (prev_seqnum(4)+1==prev_seqnum(3) && ...                                % if all 4 values are an increment of each other in the correct order
        prev_seqnum(3)+1==prev_seqnum(2) && ...
        prev_seqnum(2)+1==prev_seqnum(1) )
    
    seqnum_lock = prev_seqnum(1);                                          % set the lock to the current sequence number
    seqnum_countenable = 1;                                                % set the count enable to allow the lock signal to increment
end
if seqnum_countenable == 1                                                 % if lock enable signal is high
    seqnum_lock = seqnum_lock+1;                                           % increment the lock signal
end

%-------------------------------------------------------------------------%
% Extract and convert the header fields to decimal values

% obtain the sequence number stored in the current frame
sequence_num = bi2de(double(img_rx(seq_num_pos:seq_num_pos+seq_num_bit_len-1)'),'left-msb');

% obtain the header length — used to determine payload location
header_len = bi2de(double(img_rx(header_len_pos:header_len_pos+header_bit_len-1)'),'left-msb');

if header_len ~= 76                                                        % if header length has been recovered with errors, set to a default value
    header_len = 76;
end

% obtain the payload length — used to recover the image data in the frame
payload_len = bi2de(double(img_rx(payload_len_pos:payload_len_pos+payload_bit_len-1)'),'left-msb');

if payload_len ~= 924                                                      % if payload length has been recovered with errors, set to a default value
    payload_len = 924;
end

% obtain the padding length — used to calculate data length
padding_len = bi2de(double(img_rx(pad_len_pos:pad_len_pos+pad_bit_len-1)'),'left-msb');

% calculate data length from other header fields
data_len = payload_len - padding_len;

if data_len ~= 800                                                         % if data length has been recovered with errors, set to a default value
    data_len = 800;
end
%-------------------------------------------------------------------------%
% Find data positions and extract data from current frame

data_start = header_len+1;                                                 % find data start
data_end = header_len+data_len;                                            % find data end
data = img_rx(data_start:data_end);                                        % extract data from frame

%-------------------------------------------------------------------------%
% Search for the first valid frame

% display the information message before a frame is found
if initial_op_flag == 0
    disp('Searching for first frame...');
    initial_op_flag = 1;
end

% if sequence number is out of normal bounds
if sequence_num < 1 || sequence_num > 100                                  % sequence numbers should be between 1 & 100 for 100 column images
    if seqnum_countenable == 1                                             % if count enable for lock is high
        sequence_num = seqnum_lock;                                        % allow sequence number to be obtained from sequence number lock
    else
        valid_seq_num  = 0;                                                % if the count enable is low and hence not locked, don't recover the frame
    end
end

%-------------------------------------------------------------------------%
% If the conditions are met, extract pixel data to decimal image column

pixel_column = zeros(1,img_pixels_y);                                      % declare variable for data storage

if valid_seq_num == 1 && seqnum_lock < 100                                 % if the recovered sequence number is value and sequence number lock is less than end of frame
    disp([' Picture Column Number: ',num2str(sequence_num)]);              % indicate in command window which column has just been received using current sequence number
    
    % recover each pixel of the column from the data
    for count = 1:1:img_pixels_y
        pixel_binary = data((((count-1)*binary_len)+1):binary_len*count);  % use 'count' to extract one byte per pixel
        pixel_column(count) = bi2de(double(pixel_binary'),'left-msb');             % store decimal value of pixel in column
    end
    
    % check if the current frame (column) has been received before or not
    if seq_num_storage(sequence_num) == 0
        seq_num_storage(sequence_num) = sequence_num;                      % if not, record sequence number
        image(:,sequence_num) = pixel_column;                              % save received column of pixels into image variable using current sequence number
    end
end
if valid_seq_num == 0
    valid_seq_num = 1;                                                     % reset valid_seq_num if it has been set low
end

% if 100 frames have been received and processed
if seqnum_lock >= 100
    
    assignin('base', 'image', image);                                      % save image to MATLAB workspace
    set_param(bdroot, 'SimulationCommand', 'pause')                        % pause simulation to run plotting callback
    
    % *callback runs, then model execution continued*
    
    % reset persistent variables
    seq_num_storage = zeros(1,100);
    %image = zeros(100,100);
    image(1:100,1:100) = uint8(255);
    seqnum_lock = 0;
    seqnum_countenable = 0;
    prev_seqnum = zeros(1,4);
end
%-------------------------------------------------------------------------%
end
